simulink model "diff_drive_sim"  (R2018b)
settings: Solver=VariableStepAuto  StartTime=0.0  StopTime=489.5  RelTol=1e-3
values from neighbouring files (symbols this model uses):
  theta0 = atan2(ppval(fnder(sy,1), 0), ppval(fnder(sx,1), 0))    [diff_drive.m]
  x0 = xwp(1)    [diff_drive.m]
  y0 = ywp(1)    [diff_drive.m]
undefined symbols (not defined in the file or in its folder): breaks, xc, xdc, xddc, yc, ydc, yddc
libraries: simulink x1
settings Model: Creator=olivier  LastModifiedBy=olivier
settings SolverCC: ZeroCrossAlgorithm=Adaptive
settings DebuggingCC: MaskedZcDiagnostic=none

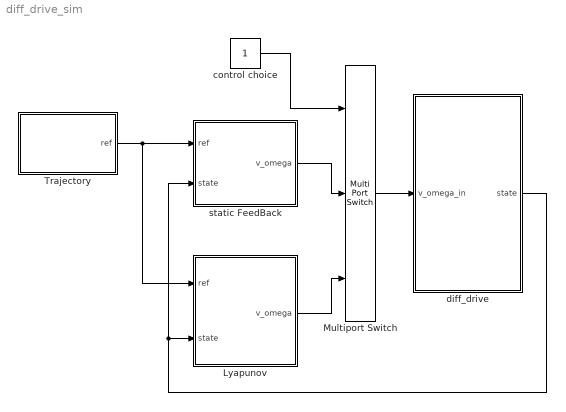
== system diff_drive_sim ==
  Lyapunov : Subsystem
  Multiport Switch : MultiPortSwitch  Inputs=2
  Trajectory : Subsystem  TreatAsAtomicUnit=on
  control choice : Constant
  diff_drive : Subsystem  mask{base=0.5, base_error=0, radius=0.2, radius_error=0, omega_max=80}
      mask prompts: base_error "Base error in percent"; radius_error "Radius error in percent"; omega_max "Wheel Max Velocity"
  static FeedBack : Subsystem
  wires:
  Trajectory/1(ref) -> Lyapunov/1(ref), static FeedBack/1(ref)
  static FeedBack/1(v_omega) -> Multiport Switch/2
  Multiport Switch/1 -> diff_drive/1(v_omega_in)
  control choice/1 -> Multiport Switch/1
  diff_drive/1(state) -> Lyapunov/2(state), static FeedBack/2(state)
  Lyapunov/1(v_omega) -> Multiport Switch/3

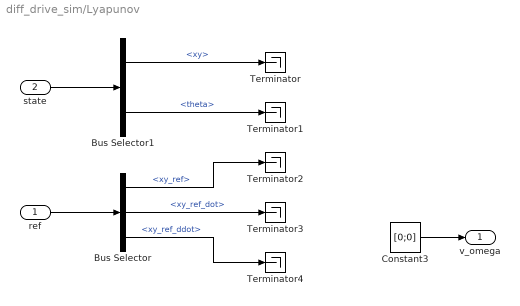
== system diff_drive_sim/Lyapunov ==
  ref : Inport
  state : Inport  Port=2
  Bus Selector : BusSelector  OutputSignals=xy_ref,xy_ref_dot,xy_ref_ddot
  Bus Selector1 : BusSelector  OutputSignals=xy,theta
  Constant3 : Constant  Value=[0;0]
  Terminator{,1..4} (5 alike) : Terminator
  v_omega : Outport
  wires:
  Constant3/1 -> v_omega/1
  ref/1 -> Bus Selector/1
  state/1 -> Bus Selector1/1
  Bus Selector/2 -> Terminator3/1  "<xy_ref_dot>"
  Bus Selector/1 -> Terminator2/1  "<xy_ref>"
  Bus Selector/3 -> Terminator4/1  "<xy_ref_ddot>"
  Bus Selector1/1 -> Terminator/1  "<xy>"
  Bus Selector1/2 -> Terminator1/1  "<theta>"

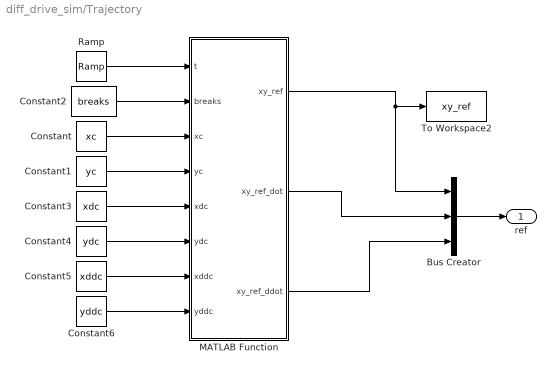
== system diff_drive_sim/Trajectory ==
  Bus Creator : BusCreator  Inputs=3
  Constant : Constant  Value=xc  VectorParams1D=off
  Constant1 : Constant  Value=yc  VectorParams1D=off
  Constant2 : Constant  Value=breaks  VectorParams1D=off
  Constant3 : Constant  Value=xdc  VectorParams1D=off
  Constant4 : Constant  Value=ydc  VectorParams1D=off
  Constant5 : Constant  Value=xddc  VectorParams1D=off
  Constant6 : Constant  Value=yddc  VectorParams1D=off
  MATLAB Function : MATLAB Function  TreatAsAtomicUnit=on
  Ramp : simulink/Sources/Ramp  slope=1  start=0  InitialOutput=0
  To Workspace2 : ToWorkspace  VariableName=xy_ref  SampleTime=-1
      settings: Save2DSignal=2-D array (concatenate along first dimension)
  ref : Outport
  wires:
  Ramp/1 -> MATLAB Function/1(t)
  MATLAB Function/1(xy_ref) -> Bus Creator/1, To Workspace2/1
  Constant3/1 -> MATLAB Function/5(xdc)
  Constant4/1 -> MATLAB Function/6(ydc)
  Constant/1 -> MATLAB Function/3(xc)
  Constant2/1 -> MATLAB Function/2(breaks)
  Constant1/1 -> MATLAB Function/4(yc)
  Constant5/1 -> MATLAB Function/7(xddc)
  Constant6/1 -> MATLAB Function/8(yddc)
  MATLAB Function/2(xy_ref_dot) -> Bus Creator/2
  MATLAB Function/3(xy_ref_ddot) -> Bus Creator/3
  Bus Creator/1 -> ref/1

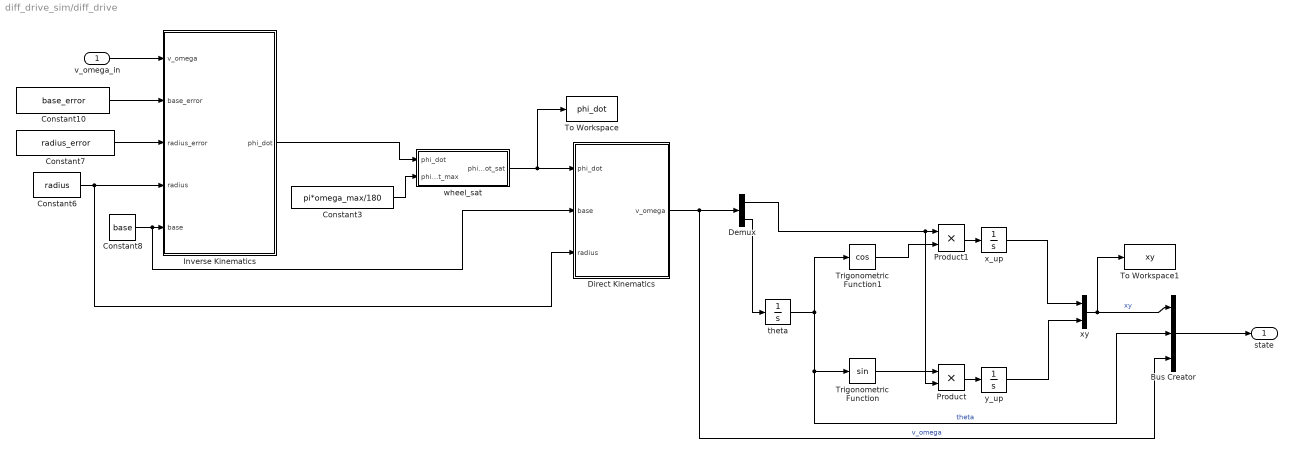
== system diff_drive_sim/diff_drive ==
  v_omega_in : Inport
  Bus Creator : BusCreator  Inputs=3
  Constant10 : Constant  Value=base_error
  Constant3 : Constant  Value=pi*omega_max/180
  Constant6 : Constant  Value=radius
  Constant7 : Constant  Value=radius_error
  Constant8 : Constant  Value=base
  Demux : Demux  Outputs=2
  Direct Kinematics : MATLAB Function  TreatAsAtomicUnit=on
  Inverse Kinematics : MATLAB Function  TreatAsAtomicUnit=on
  Product : Product
  Product1 : Product
  To Workspace : ToWorkspace  VariableName=phi_dot  SampleTime=-1
      settings: Save2DSignal=2-D array (concatenate along first dimension)
  To Workspace1 : ToWorkspace  VariableName=xy  SampleTime=-1
      settings: Save2DSignal=2-D array (concatenate along first dimension)
  Trigonometric Function : Trigonometry
  Trigonometric Function1 : Trigonometry  Operator=cos
  theta : Integrator  InitialCondition=theta0
  wheel_sat : Subsystem
  x_up : Integrator  InitialCondition=x0
  xy : Mux  Inputs=2
  y_up : Integrator  InitialCondition=y0
  state : Outport
  wires:
  theta/1 -> Trigonometric Function1/1, Trigonometric Function/1, Bus Creator/2  "theta"
  Trigonometric Function1/1 -> Product1/2
  Trigonometric Function/1 -> Product/1
  Product/1 -> y_up/1
  Product1/1 -> x_up/1
  x_up/1 -> xy/1
  Constant3/1 -> wheel_sat/2(phi_dot_max)
  Direct Kinematics/1(v_omega) -> Bus Creator/3, Demux/1  "v_omega"
  Demux/1 -> Product/2, Product1/1
  Demux/2 -> theta/1
  y_up/1 -> xy/2
  wheel_sat/1(phi_dot_sat) -> Direct Kinematics/1(phi_dot), To Workspace/1
  xy/1 -> Bus Creator/1, To Workspace1/1  "xy"
  Bus Creator/1 -> state/1
  Inverse Kinematics/1(phi_dot) -> wheel_sat/1(phi_dot)
  v_omega_in/1 -> Inverse Kinematics/1(v_omega)
  Constant10/1 -> Inverse Kinematics/2(base_error)
  Constant7/1 -> Inverse Kinematics/3(radius_error)
  Constant6/1 -> Inverse Kinematics/4(radius), Direct Kinematics/3(radius)
  Constant8/1 -> Direct Kinematics/2(base), Inverse Kinematics/5(base)

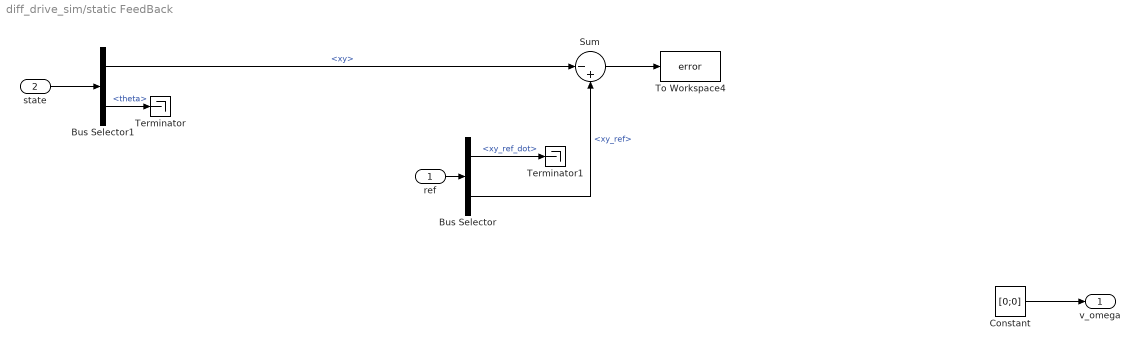
== system diff_drive_sim/static FeedBack ==
  ref : Inport
  state : Inport  Port=2
  Bus Selector : BusSelector  OutputSignals=xy_ref_dot,xy_ref
  Bus Selector1 : BusSelector  OutputSignals=xy,theta
  Constant : Constant  Value=[0;0]
  Sum : Sum  Inputs=|-+
  Terminator : Terminator
  Terminator1 : Terminator
  To Workspace4 : ToWorkspace  VariableName=error  SampleTime=-1
      settings: Save2DSignal=2-D array (concatenate along first dimension)
  v_omega : Outport
  wires:
  ref/1 -> Bus Selector/1
  state/1 -> Bus Selector1/1
  Bus Selector/2 -> Sum/2  "<xy_ref>"
  Bus Selector1/1 -> Sum/1  "<xy>"
  Sum/1 -> To Workspace4/1
  Constant/1 -> v_omega/1
  Bus Selector1/2 -> Terminator/1  "<theta>"
  Bus Selector/1 -> Terminator1/1  "<xy_ref_dot>"

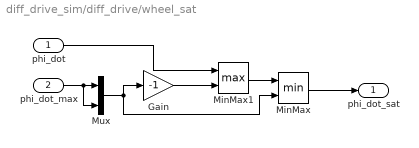
== system diff_drive_sim/diff_drive/wheel_sat ==
  phi_dot : Inport
  phi_dot_max : Inport  Port=2
  Gain : Gain  Gain=-1
  MinMax : MinMax  Inputs=2
  MinMax1 : MinMax  Function=max  Inputs=2
  Mux : Mux  Inputs=2
  phi_dot_sat : Outport
  wires:
  Gain/1 -> MinMax1/2
  MinMax/1 -> phi_dot_sat/1
  phi_dot_max/1 -> Mux/2, Mux/1
  phi_dot/1 -> MinMax1/1
  MinMax1/1 -> MinMax/1
  Mux/1 -> MinMax/2, Gain/1

== matlab function diff_drive_sim/diff_drive/Inverse Kinematics ==
  data: v_omega input; base_error input; radius_error input; radius input; phi_dot output; base input
function phi_dot = ik(v_omega, base_error, radius_error, radius, base)

base = base * (1+base_error*0.01);
radius = radius * (1+radius_error*0.01);

phi_dot = [(v_omega(1)+base*v_omega(2))/radius; (v_omega(1)-base*v_omega(2))/radius];

== matlab function diff_drive_sim/Trajectory/MATLAB Function ==
  data: xy_ref output; t input; breaks input; xc input; yc input; xy_ref_dot output; xy_ref_ddot output; xdc input; ydc input; xddc input; yddc input
function [xy_ref, xy_ref_dot, xy_ref_ddot] = reference(t, breaks, xc, yc, xdc, ydc, xddc, yddc)

sx = mkpp(breaks, xc);
sy = mkpp(breaks, yc);


if t > sx.breaks(end)
    t = sx.breaks(end);
    xy_ref_dot = [0; 0];
    xy_ref_ddot = [0; 0];
else
    xy_ref_dot = [ppval(mkpp(breaks, xdc), t); ppval(mkpp(breaks, ydc), t)];
    xy_ref_ddot = [ppval(mkpp(breaks, xddc), t); ppval(mkpp(breaks, yddc), t)];
end
xy_ref = [ppval(sx, t); ppval(sy, t)];

== matlab function diff_drive_sim/diff_drive/Direct Kinematics ==
  data: phi_dot input; v_omega output; base input; radius input
function v_omega = dk(phi_dot, base, radius)

v_omega = [radius*(phi_dot(1)+phi_dot(2))/2; radius*(phi_dot(1)-phi_dot(2))/(2*base)];
